simulink model "Boost_PFC_BayesOpt_v1_WORKING_BASELINE"  (R2025a)
settings: Solver=FixedStepDiscrete  StartTime=0.0  StopTime=2  FixedStep=1e-7  RelTol=1e-3
libraries: spsSeriesRLCBranchLib x4, spsVoltageMeasurementLib x3, spsParallelRLCBranchLib x2, spsACVoltageSourceLib x1, spsDiodeLib x1, spsGroundLib x1, spsIGBTLib x1, spsCurrentMeasurementLib x1, spsMosfetLib x1, spsUniversalBridgeLib x1, sps_lib x1
settings Model: Creator=ahmet  LastModifiedBy=ahmet

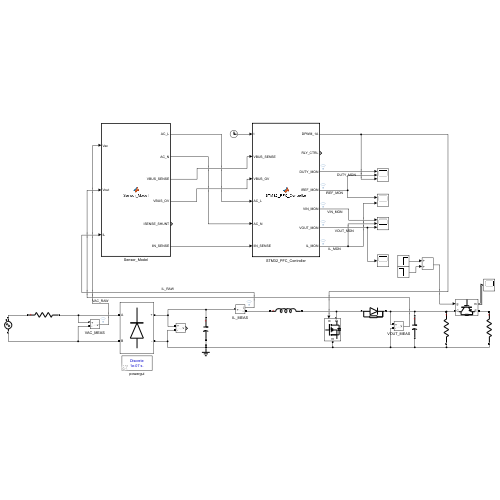
[thumbnail: Simulink's stored preview of the top-level diagram]
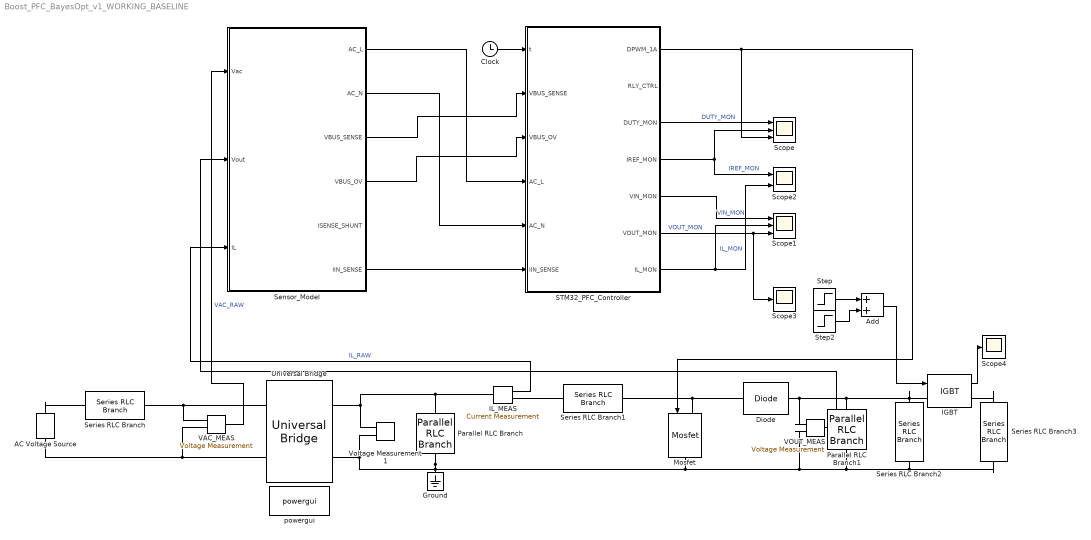
== system Boost_PFC_BayesOpt_v1_WORKING_BASELINE ==
  AC Voltage Source : spsACVoltageSourceLib/AC Voltage Source  Amplitude=325  Phase=0  Frequency=50  SampleTime=0  Measurements=None  BusType=swing  Pref=10e3  Qref=0  Qmin=-inf  Qmax=+inf
  Add : Sum
  Clock : Clock
  Diode : spsDiodeLib/Diode  Ron=0.001  Lon=0  Vf=0.8  IC=0  UseSnubber=0  Rs=1e5  Cs=inf  Measurements=off
  Ground : spsGroundLib/Ground  LConnTagsString=a
  IGBT : spsIGBTLib/IGBT  Ron=0.001  Lon=0  Vf=1  Tf=1e-6  Tt=2e-6  IC=0  Rs=1e5  Cs=inf  Measurements=on
  IL_MEAS : spsCurrentMeasurementLib/Current Measurement  PhasorSimulation=off  OutputType=Complex  PSBequivalent=0
  Mosfet : spsMosfetLib/Mosfet  Ron=0.19  Lon=0  Rd=0.01  Vfd=0.9  IC=0  Rs=1e5  Cs=inf  Measurements=off
  Parallel RLC Branch : spsParallelRLCBranchLib/Parallel RLC Branch  LConnTagsString=a  RConnTagsString=__new0  BranchType=C  Resistance=1  Inductance=1e-3  SetiL0=off  InitialCurrent=0  Capacitance=1e-6  Setx0=off  InitialVoltage=0  Measurements=None
  Parallel RLC Branch1 : spsParallelRLCBranchLib/Parallel RLC Branch  LConnTagsString=a  RConnTagsString=__new0  BranchType=C  Resistance=1  Inductance=1e-3  SetiL0=off  InitialCurrent=0  Capacitance=1360e-6  Setx0=off  InitialVoltage=0  Measurements=None
  STM32_PFC_Controller : MATLAB Function  TreatAsAtomicUnit=on
  Scope : Scope  NumInputPorts=3
      settings: ActiveDisplayYMinimum=-0.10554957085863778  ActiveDisplayYMaximum=0.94994613772774028  DataLoggingVariableName=ScopeData2
  Scope1 : Scope  NumInputPorts=3
      settings: ActiveDisplayYMinimum=-40.624879495450678  ActiveDisplayYMaximum=365.62391545905615
  Scope2 : Scope  NumInputPorts=2
      settings: ActiveDisplayYMinimum=-1.5851546899227209  ActiveDisplayYMaximum=11.843949047221777
  Scope3 : Scope
      settings: ActiveDisplayYMinimum=314.05537103883637  ActiveDisplayYMaximum=430.29627915318162  DataLoggingVariableName=ScopeData3
  Scope4 : Scope
      settings: ActiveDisplayYMinimum=-53.682455031069871  ActiveDisplayYMaximum=483.14209527962896  DataLoggingVariableName=ScopeData4
  Sensor_Model : MATLAB Function  TreatAsAtomicUnit=on
  Series RLC Branch : spsSeriesRLCBranchLib/Series RLC Branch  LConnTagsString=__new0  RConnTagsString=__new0  BranchType=R  Resistance=0.1  Inductance=1e-3  SetiL0=off  InitialCurrent=0  Capacitance=1e-6  Setx0=off  InitialVoltage=0  Measurements=None
  Series RLC Branch1 : spsSeriesRLCBranchLib/Series RLC Branch  LConnTagsString=__new0  RConnTagsString=__new0  BranchType=L  Resistance=1  Inductance=311e-6  SetiL0=off  InitialCurrent=0  Capacitance=1e-6  Setx0=off  InitialVoltage=0  Measurements=None
  Series RLC Branch2 : spsSeriesRLCBranchLib/Series RLC Branch  LConnTagsString=__new0  RConnTagsString=__new0  BranchType=R  Resistance=533.3  Inductance=1e-3  SetiL0=off  InitialCurrent=0  Capacitance=1e-6  Setx0=off  InitialVoltage=0  Measurements=None
  Series RLC Branch3 : spsSeriesRLCBranchLib/Series RLC Branch  LConnTagsString=__new0  RConnTagsString=__new0  BranchType=R  Resistance=145  Inductance=1e-3  SetiL0=off  InitialCurrent=0  Capacitance=1e-6  Setx0=off  InitialVoltage=0  Measurements=None
  Step : Step  Time=0.6  SampleTime=0
  Step2 : Step  After=-1  SampleTime=0
  Universal Bridge : spsUniversalBridgeLib/Universal Bridge  Arms=2  SnubberResistance=1e5  SnubberCapacitance=inf  Device=Diodes  Ron=1e-3  Lon=0  ForwardVoltages="[  0  0  ]"  ForwardVoltage=0.9  GTOparameters=[ 10e-6 , 20e-6 ]  IGBTparameters=[ 1e-6 , 2e-6 ]  Measurements=None  Measurements_2=None  converterType=Rectifier
  VAC_MEAS : spsVoltageMeasurementLib/Voltage Measurement  PhasorSimulation=off  OutputType=Complex  PSBequivalent=0
  VOUT_MEAS : spsVoltageMeasurementLib/Voltage Measurement  PhasorSimulation=off  OutputType=Complex  PSBequivalent=0
  Voltage Measurement1 : spsVoltageMeasurementLib/Voltage Measurement  PhasorSimulation=off  OutputType=Complex  PSBequivalent=0
  powergui : sps_lib/powergui  Priority=1  SimulationMode=Discrete  SampleTime=1e-7  frequency=60  Iterations=50  frequencyindice=50  Pbase=100e6  ErrMax=1e-4  UnitsV=kV  UnitsW=MW  buscounter=0  FunctionMessages=off  echomessages=off  EnableUseOfTLC=off  CurrentSourceSwitches=off  DisableSnubberDevices=off  DisableRonSwitches=off  DisableVfSwitches=off  DisplayEquations=off  AutomaticDiscreteSolvers=off  SolverType=Tustin/Backward Euler (TBE)  Interpol=off  ExternalGateDelay=off  methode=off  Ts=100  x0status=blocks  SPID=on  SwTol=0  HookPort=off  NonlinearTolerance=1e-4  nMaxIteration=100  ContinueOnMaxIteration=off  RestoreLinks=warning  ResistiveCurrentMeasurement=off  Frange=[0:2:500]  Ylog=off  Xlog=on  ShowGrid=off  save=off  variable=ZData  structure=0  ZoomFFT=off  StartTime=0.0  cycles=1  DisplayStyle=1  fundamental=60  FreqAxis=off  MaxFrequency=1000  frequencyindicesteady=1  RmsSteady=1  display=off
  wires:
  STM32_PFC_Controller/1(DPWM_1A) -> Mosfet/1, Scope/3
  Clock/1 -> STM32_PFC_Controller/1(t)
  Sensor_Model/3(VBUS_SENSE) -> STM32_PFC_Controller/2(VBUS_SENSE)
  Sensor_Model/4(VBUS_OV) -> STM32_PFC_Controller/3(VBUS_OV)
  Sensor_Model/1(AC_L) -> STM32_PFC_Controller/4(AC_L)
  Sensor_Model/2(AC_N) -> STM32_PFC_Controller/5(AC_N)
  VAC_MEAS/1 -> Sensor_Model/1(Vac)  "VAC_RAW"
  VOUT_MEAS/1 -> Sensor_Model/2(Vout)
  IL_MEAS/1 -> Sensor_Model/3(IL)  "IL_RAW"
  Sensor_Model/6(IIN_SENSE) -> STM32_PFC_Controller/6(IIN_SENSE)
  STM32_PFC_Controller/7(IL_MON) -> Scope2/2, Scope1/2  "IL_MON"
  STM32_PFC_Controller/6(VOUT_MON) -> Scope3/1, Scope1/3  "VOUT_MON"
  STM32_PFC_Controller/5(VIN_MON) -> Scope1/1  "VIN_MON"
  STM32_PFC_Controller/4(IREF_MON) -> Scope2/1, Scope/2  "IREF_MON"
  STM32_PFC_Controller/3(DUTY_MON) -> Scope/1  "DUTY_MON"
  Step/1 -> Add/1
  Step2/1 -> Add/2
  Add/1 -> IGBT/1
  IGBT/1 -> Scope4/1
  connections:
  AC Voltage Source/RConn1 -- Series RLC Branch/LConn1
  Series RLC Branch/RConn1 -- VAC_MEAS/LConn1 -- Universal Bridge/LConn1
  AC Voltage Source/LConn1 -- VAC_MEAS/LConn2 -- Universal Bridge/LConn2
  Voltage Measurement1/LConn1 -- Parallel RLC Branch/LConn1 -- IL_MEAS/LConn1 -- Universal Bridge/RConn1
  Parallel RLC Branch/RConn1 -- VOUT_MEAS/LConn2 -- Series RLC Branch3/RConn1 -- Series RLC Branch2/RConn1 -- Parallel RLC Branch1/RConn1 -- Mosfet/RConn1 -- Voltage Measurement1/LConn2 -- Universal Bridge/RConn2 -- Ground/LConn1
  Mosfet/LConn1 -- Series RLC Branch1/RConn1 -- Diode/LConn1
  Diode/RConn1 -- VOUT_MEAS/LConn1 -- IGBT/LConn1 -- Series RLC Branch2/LConn1 -- Parallel RLC Branch1/LConn1
  IL_MEAS/RConn1 -- Series RLC Branch1/LConn1
  Series RLC Branch3/LConn1 -- IGBT/RConn1

== matlab function Boost_PFC_BayesOpt_v1_WORKING_BASELINE/STM32_PFC_Controller ==
  data: t input; DPWM_1A output; VBUS_SENSE input; VBUS_OV input; RLY_CTRL output; DUTY_MON output; IREF_MON output; VIN_MON output; VOUT_MON output; AC_L input; AC_N input; IIN_SENSE input; IL_MON output
function [DPWM_1A, RLY_CTRL, DUTY_MON, IREF_MON, ...
          VIN_MON, VOUT_MON, IL_MON] = ...
          STM32_PFC_Controller(t, VBUS_SENSE, VBUS_OV, ...
          AC_L, AC_N, IIN_SENSE)

% =========================================================
% GENERAL CONSTANTS
% =========================================================

FSW = 75e3;
TSW = 1.0 / FSW;

PWM_START = 0.05;
SOFT_TIME = 0.20;

VOUT_START  = 330.0;
VOUT_TARGET = 400.0;
VOUT_OVP    = 430.0;

DUTY_MIN    = 0.0;
DUTY_MAX    = 0.85;
DUTY_FF_MAX = 0.75;

IAMP_MAX = 14.0;
IL_SW_LIMIT = 18.0;

I_INT_MIN = -0.35;
I_INT_MAX =  0.35;

% =========================================================
% ZERO-CROSSING CONTROL
% =========================================================

VIN_PWM_OFF = 10.0;
VIN_RAMP_END = 50.0;

VIN_PEAK_NOM = 230.0 * sqrt(2.0);

% =========================================================
% CYCLE-BY-CYCLE PEAK-CURRENT CONTROL
% =========================================================

I_PEAK_MIN = 1.2;
I_PEAK_MARGIN = 1.3;

% =========================================================
% SENSOR-SCALING CONSTANTS
% =========================================================

K_VBUS = 3.16e3 / (600e3 + 3.16e3);
K_AC   = 3.6e3  / (600e3 + 3.6e3);

RSHUNT = 0.008;
GAIN_I = 21.1;

% =========================================================
% PI-CONTROLLER GAINS
% =========================================================
% Gains are defined directly in the code.
% No Workspace or Symbols Pane setting is required.

KP_V = 0.010;
KI_V = 0.80;

KP_I = 0.018;
KI_I = 75.0;

% =========================================================
% PERSISTENT CONTROLLER STATES
% =========================================================

persistent last_period
persistent v_int
persistent i_int
persistent duty_mem
persistent iref_mem

persistent peak_trip
persistent peak_limit_mem

if isempty(last_period)

    last_period = -1.0;

    v_int = 0.0;
    i_int = 0.0;

    duty_mem = 0.0;
    iref_mem = 0.0;

    peak_trip = false;
    peak_limit_mem = I_PEAK_MIN;

end

% =========================================================
% CONVERT SENSOR SIGNALS TO PHYSICAL VALUES
% =========================================================

vout = VBUS_SENSE / K_VBUS;
vov  = VBUS_OV / K_VBUS;

vac_scaled = AC_L - AC_N;
vin = abs(vac_scaled / K_AC);

il = IIN_SENSE / (RSHUNT * GAIN_I);
il = abs(il);

% =========================================================
% DEFAULT OUTPUTS
% =========================================================

DPWM_1A = 0.0;
RLY_CTRL = 0.0;

DUTY_MON = duty_mem;
IREF_MON = iref_mem;

VIN_MON  = vin;
VOUT_MON = vout;
IL_MON   = il;

% =========================================================
% RELAY CONTROL
% =========================================================

if t >= 0.02
    RLY_CTRL = 1.0;
else
    RLY_CTRL = 0.0;
end

% =========================================================
% BEFORE PWM START
% =========================================================

if t < PWM_START

    last_period = -1.0;

    v_int = 0.0;
    i_int = 0.0;

    duty_mem = 0.0;
    iref_mem = 0.0;

    peak_trip = false;
    peak_limit_mem = I_PEAK_MIN;

    DPWM_1A = 0.0;

    DUTY_MON = 0.0;
    IREF_MON = 0.0;

    VIN_MON  = vin;
    VOUT_MON = vout;
    IL_MON   = il;

    return;
end

% Time measured from PWM activation
t_pwm = t - PWM_START;

% Current PWM-period number
period_now = floor(t_pwm / TSW);

% =========================================================
% CONTROL UPDATE ONCE PER SWITCHING PERIOD
% =========================================================

if period_now ~= last_period

    last_period = period_now;

    % Reset cycle-by-cycle current trip
    peak_trip = false;

    % -----------------------------------------------------
    % SOFT-START VOLTAGE REFERENCE
    % -----------------------------------------------------

    if t_pwm < SOFT_TIME

        vref = VOUT_START + ...
            (VOUT_TARGET - VOUT_START) * ...
            (t_pwm / SOFT_TIME);

    else

        vref = VOUT_TARGET;

    end

    % -----------------------------------------------------
    % ZERO-CROSSING RAMP FACTOR
    % -----------------------------------------------------

    if vin <= VIN_PWM_OFF

        zc_gain = 0.0;

    elseif vin >= VIN_RAMP_END

        zc_gain = 1.0;

    else

        zc_gain = (vin - VIN_PWM_OFF) / ...
                  (VIN_RAMP_END - VIN_PWM_OFF);

    end

    % -----------------------------------------------------
    % OUTER VOLTAGE PI LOOP
    % -----------------------------------------------------

    ev = vref - vout;

    i_amp_unsat = KP_V * ev + v_int;

    % Conditional-integration anti-windup
    if ~((i_amp_unsat >= IAMP_MAX && ev > 0.0) || ...
         (i_amp_unsat <= 0.0 && ev < 0.0))

        v_int = v_int + KI_V * ev * TSW;

    end

    % Voltage integrator limits
    if v_int > IAMP_MAX
        v_int = IAMP_MAX;
    elseif v_int < 0.0
        v_int = 0.0;
    end

    % Recalculate output after integrator update
    i_amp = KP_V * ev + v_int;

    if i_amp > IAMP_MAX
        i_amp = IAMP_MAX;
    elseif i_amp < 0.0
        i_amp = 0.0;
    end

    % -----------------------------------------------------
    % SINUSOIDAL CURRENT-REFERENCE GENERATION
    % -----------------------------------------------------

    vin_norm = vin / VIN_PEAK_NOM;

    if vin_norm > 1.0
        vin_norm = 1.0;
    elseif vin_norm < 0.0
        vin_norm = 0.0;
    end

    iref = i_amp * vin_norm * zc_gain;

    % -----------------------------------------------------
    % BOOST DUTY FEED-FORWARD
    % -----------------------------------------------------

    if vout > 100.0
        duty_ff_raw = 1.0 - vin / vout;
    else
        duty_ff_raw = 0.20;
    end

    if duty_ff_raw > DUTY_FF_MAX
        duty_ff_raw = DUTY_FF_MAX;
    elseif duty_ff_raw < 0.0
        duty_ff_raw = 0.0;
    end

    duty_ff = duty_ff_raw * zc_gain;

    % -----------------------------------------------------
    % INNER CURRENT PI LOOP
    % -----------------------------------------------------

    ei = iref - il;

    duty_unsat = duty_ff + KP_I * ei + i_int;

    % Conditional-integration anti-windup
    if ~((duty_unsat >= DUTY_MAX && ei > 0.0) || ...
         (duty_unsat <= DUTY_MIN && ei < 0.0))

        i_int = i_int + KI_I * ei * TSW;

    end

    % Current integrator limits
    if i_int > I_INT_MAX
        i_int = I_INT_MAX;
    elseif i_int < I_INT_MIN
        i_int = I_INT_MIN;
    end

    % Recalculate duty after integrator update
    duty_unsat = duty_ff + KP_I * ei + i_int;

    if duty_unsat > DUTY_MAX
        duty = DUTY_MAX;
    elseif duty_unsat < DUTY_MIN
        duty = DUTY_MIN;
    else
        duty = duty_unsat;
    end

    % -----------------------------------------------------
    % PWM-OFF REGION AROUND ZERO CROSSING
    % -----------------------------------------------------

    if vin <= VIN_PWM_OFF

        duty = 0.0;
        iref = 0.0;

        i_int = 0.0;

    end

    % -----------------------------------------------------
    % OVERVOLTAGE PROTECTION
    % -----------------------------------------------------

    if vout >= VOUT_OVP || vov >= VOUT_OVP

        duty = 0.0;
        iref = 0.0;

        i_int = 0.0;
        v_int = 0.0;

    end

    % -----------------------------------------------------
    % ABSOLUTE OVERCURRENT PROTECTION
    % -----------------------------------------------------

    if il >= IL_SW_LIMIT

        duty = 0.0;
        iref = 0.0;

        i_int = 0.0;
        peak_trip = true;

    end

    % -----------------------------------------------------
    % PEAK-CURRENT LIMIT FOR CURRENT PWM PERIOD
    % -----------------------------------------------------

    peak_limit = iref + I_PEAK_MARGIN;

    if peak_limit < I_PEAK_MIN
        peak_limit = I_PEAK_MIN;
    elseif peak_limit > IL_SW_LIMIT
        peak_limit = IL_SW_LIMIT;
    end

    peak_limit_mem = peak_limit;

    duty_mem = duty;
    iref_mem = iref;

end

% =========================================================
% CURRENT PWM POSITION
% =========================================================

t_pwm = t - PWM_START;
tau = t_pwm - floor(t_pwm / TSW) * TSW;

if tau < duty_mem * TSW
    pwm_window = true;
else
    pwm_window = false;
end

% =========================================================
% CYCLE-BY-CYCLE PEAK-CURRENT CUTOFF
% =========================================================

if pwm_window && il >= peak_limit_mem
    peak_trip = true;
end

% =========================================================
% FAST ABSOLUTE PROTECTION
% =========================================================

if vout >= VOUT_OVP || vov >= VOUT_OVP

    duty_mem = 0.0;
    iref_mem = 0.0;

    i_int = 0.0;
    v_int = 0.0;

    peak_trip = true;

end

if il >= IL_SW_LIMIT

    duty_mem = 0.0;
    iref_mem = 0.0;

    i_int = 0.0;

    peak_trip = true;

end

% =========================================================
% DIGITAL PWM GENERATION
% =========================================================

if (tau < duty_mem * TSW) && (~peak_trip)
    DPWM_1A = 1.0;
else
    DPWM_1A = 0.0;
end

% =========================================================
% MONITOR OUTPUTS
% =========================================================

DUTY_MON = duty_mem;
IREF_MON = iref_mem;

VIN_MON  = vin;
VOUT_MON = vout;
IL_MON   = il;

end

== matlab function Boost_PFC_BayesOpt_v1_WORKING_BASELINE/Sensor_Model ==
  data: Vac input; AC_L output; Vout input; IL input; AC_N output; VBUS_SENSE output; VBUS_OV output; ISENSE_SHUNT output; IIN_SENSE output
function [AC_L, AC_N, VBUS_SENSE, VBUS_OV, ...
          ISENSE_SHUNT, IIN_SENSE] = Sensor_Model(Vac, Vout, IL)

% =========================================================
% SENSOR MODEL
% =========================================================

ADC_MAX = 3.3;

% DC-bus voltage-divider ratio
K_VBUS = 3.16e3 / (600e3 + 3.16e3);

% AC-input voltage-divider ratio
K_AC = 3.6e3 / (600e3 + 3.6e3);

% Current-sensing parameters
RSHUNT = 0.008;
GAIN_I = 21.1;

% =========================================================
% AC INPUT-VOLTAGE SENSING
% =========================================================

% Both ADC signals remain positive.
if Vac >= 0.0
    AC_L = Vac * K_AC;
    AC_N = 0.0;
else
    AC_L = 0.0;
    AC_N = (-Vac) * K_AC;
end

% ADC saturation
if AC_L > ADC_MAX
    AC_L = ADC_MAX;
elseif AC_L < 0.0
    AC_L = 0.0;
end

if AC_N > ADC_MAX
    AC_N = ADC_MAX;
elseif AC_N < 0.0
    AC_N = 0.0;
end

% =========================================================
% DC-BUS VOLTAGE SENSING
% =========================================================

VBUS_SENSE = Vout * K_VBUS;
VBUS_OV    = Vout * K_VBUS;

if VBUS_SENSE > ADC_MAX
    VBUS_SENSE = ADC_MAX;
elseif VBUS_SENSE < 0.0
    VBUS_SENSE = 0.0;
end

if VBUS_OV > ADC_MAX
    VBUS_OV = ADC_MAX;
elseif VBUS_OV < 0.0
    VBUS_OV = 0.0;
end

% =========================================================
% INDUCTOR-CURRENT SENSING
% =========================================================

IL_abs = abs(IL);

% Raw voltage directly across the shunt
ISENSE_SHUNT = IL_abs * RSHUNT;

% Amplified signal applied to the STM32 ADC
IIN_SENSE = IL_abs * RSHUNT * GAIN_I;

if IIN_SENSE > ADC_MAX
    IIN_SENSE = ADC_MAX;
elseif IIN_SENSE < 0.0
    IIN_SENSE = 0.0;
end

end
